simulink model "bu_abslut125_rombina_32"  (R2021b)
settings: Solver=VariableStepAuto  StartTime=0.0  StopTime=359  RelTol=1e-3
libraries: hdlBasic x1686, vmcUtilities x1
(part 4 of 8)

== matlab function bu_abslut125_rombina_32/MATLAB Function ==
  data: u input; y output; x input
function y = fcn(u,x)

y = immse(u,x);

== matlab function bu_abslut125_rombina_32/MATLAB Function2 ==
  data: x input; out output; y input
function out = fcn(x,y)
out = sqrt(x.^2 + y.^2);
